simulink model "completed_microinverter_setup"  (R2022a)
settings: Solver=FixedStepDiscrete  StartTime=0.0  StopTime=2  FixedStep=Ts  RelTol=1e-3
InitFcn:
  | Ts=1e-6;
  | Tcs=1e-4;
values from neighbouring files (symbols this model uses):
  C1_filter = 2e-6    (= 2e-06)    [q4.m]
  C_filter = 100e-6    (= 0.0001)    [q1.m]    (also in q2.m; q4.m = 2e-06)
  f_center = 50    [q4.m]
  F_switch = 1e3    (= 1000)    [q1.m]
  Ki_current = L_filter*Wn^2    (= 15791.3670417)    [q1.m]    (also in q2.m = 63165.468167; q4.m = 493.480220054)
  Ki_pll = (Wn^2) / A    (= 394784.176044)    [q1.m]    (also in q4.m = 1579136.70417)
  Ki_power = 100    [q4.m]
  Ki_voltage = C_filter*Wn^2    (= 3.55305758439)    [q1.m]    (also in q4.m = 0.0710611516878)
  Kp_current = 2*L_filter*DF*Wn    (= 110.584061406)    [q1.m]    (also in q2.m = 71.0753921948; q4.m = 5.49778714378)
  Kp_pll = 2*DF / sqrt(A/Ki_pll)    [q1.m]    (also in q4.m = 2*DF / sqrt(1/Ki_pll))
  Kp_power = 0    [q4.m]
  Kp_voltage = 2*C_filter*DF*Wn    (= 0.0565486677646)    [q1.m]    (also in q4.m = 0.00791681348705)
  L1_filter = 1.5e-3    (= 0.0015)    [q4.m]
  L2_filter = 1.0e-3    (= 0.001)    [q4.m]
  L_filter = 40e-3    (= 0.04)    [q1.m]    (also in q2.m; q4.m = 0.00125)
  L_load = sqrt((R_load * V_rms^2)/P_load - R_load^2) / w    [q1.m]    (also in q4.m)
  R_load = (V_rms^2) * (pf_load^2) / P_load    (= 43.32)    [q1.m]    (also in q4.m)
  Rd_filter = 0.2    [q4.m]
  Tes = 20*Ts    (= 2e-05)    [q1.m]    (also in q4.m)
  V_dc = sqrt(2) * sqrt(3) * V_rms    [q1.m]    (also in q4.m = V_rms * sqrt(3) * sqrt(2))
undefined symbols (not defined in the file or in its folder): DiscIntNeverNeededParam
libraries: ee_lib x111, nesl_utility x28, fl_lib x23, spsabctodq0Lib x11, dspindex x3, spsTriangleGeneratorLib x2, spsdq0toabcLib x2
(part 3 of 4)

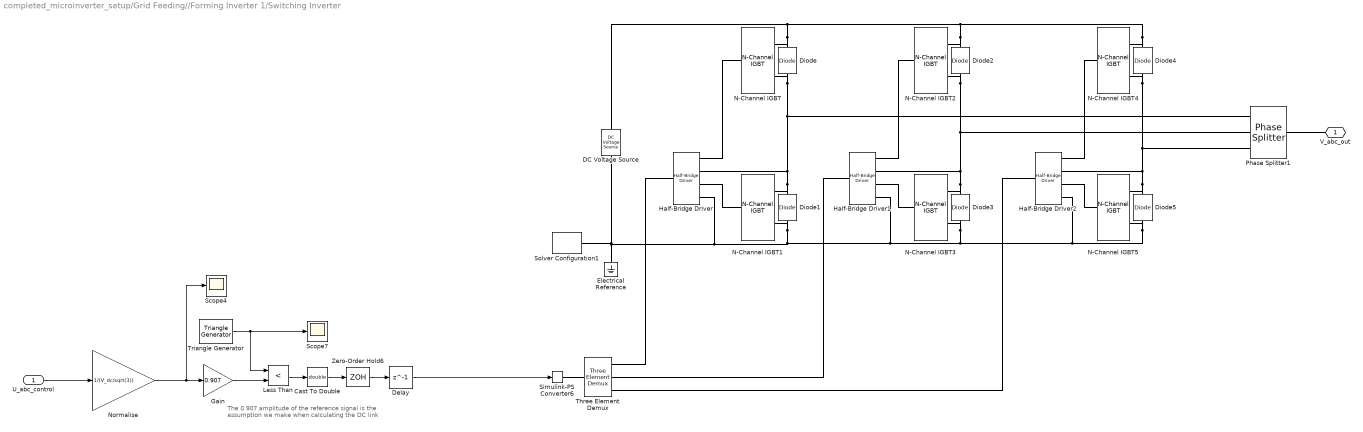
== system completed_microinverter_setup/Grid Feeding//Forming Inverter 1/Switching Inverter ==
  note: The 0.907 amplitude of the reference signal is the assumption we make when calculating the DC link
  U_abc_control : Inport
  Cast To Double : DataTypeConversion  OutDataTypeStr=double  SaturateOnIntegerOverflow=off  RndMeth=Floor
  DC Voltage Source : ee_lib/Additional Components/SPICE Sources/DC Voltage Source  DC=V_dc V
  Delay : Delay  DelayLength=1
  Diode{,1..5} (6 alike) : ee_lib/Semiconductors & Converters/Diode  ModelType=ee.enum.diode.modelType.pwl  TableType=ee.enum.diode.tableType.IfMat  IfMat=[.07, .12, .19, 1.75, 4.24, 7.32, 11.2; .16, .3, .72, 2.14, 5.02, 8.35, 13.12] A  VfMat=[.9, 1.15, 1.25, 1.5, 1.75, 2.17, 2.6, 2.85; .58, .68, .75, 1.1, 1.38, 1.77, 2.27, 2.7] V  TjVec=[25, 125] degC  VfVec=[.5, .7, .9, 1.3, 1.7, 2.1, 2.5] V  IfVec=[.1, .2, .5, 1, 2, 4, 7, 10] A  Vf=0.6 V  Ron=0.3 Ohm  Goff=1e-8 S  prmExp=ee.enum.diode.expParam.useTwo  I12=[.0137, .545] A  V12=[.6, .7] V  RS=0 Ohm  Tmeas=25 degC  IS=1e-12 A  ec=1  I1=0.0137 A  V1=0.6 V  N_series=1  N_parallel=1  Rz=0.3 Ohm  BV=inf V  C_param=ee.enum.diode.capParam.fixed  CJ=5 pF  CJ0=5 pF  Vvec=[.1, 10, 100] V  Cvec=[3.5, 1, .4] pF  VJ=1 V  Mgrad=0.5  FC=0.5  Q_param=ee.enum.diode.recoveryParam.off  iRM=-7.15 A  iF=4 A  didt=-750 A/us  trr_factor=3  trr=115 ns  Qrr=150 nA*s  Vr=-600 V  Ls=150 nH  Erec=0.03 J  TT=50 ns  tau=100 ns  T_param=ee.enum.diode.temperatureParam.off  Tdevice=25 degC  I1_T2=0.245 A  V1_T2=0.5 V  IS_T2=1.25e-7 A  Tmeas2=125 degC  XTI_param=ee.enum.diode.xtiParam.pn  XTI=3  EG_param=ee.enum.diode.egapParam.material_si  EG=1.11 eV  dBVdT=0 V/K  enable_faults=simscape.enum.onoff.off  fault_action=simscape.enum.assert.action.none  fault_types=ee.enum.diode.faults.open  tau_fault=1e-3 s  IfMat_faulted=[.07, .12, .19, 1.75, 4.24, 7.32, 11.2; .16, .3, .72, 2.14, 4.02, 6.35, 9.12] A  VfMat_faulted=[.9, 1.15, 1.25, 1.5, 1.75, 2.17, 2.6, 2.85; .58, .68, .75, 1.1, 1.38, 1.77, 2.27, 2.7] V  VfVec_faulted=[.5, .7, .9, 1.3, 1.7, 2.1, 2.5] V  IfVec_faulted=[.1, .2, .5, 1, 2, 4, 7, 10] A  Ropen_faulted=1000 Ohm  Gshort_faulted=1000 1/Ohm  Vf_faulted=0.6 V  Ron_faulted=0.3 Ohm  Goff_faulted=1e-8 S  I12_faulted=[.0137, .545] A  V12_faulted=[.6, .7] V  IS_faulted=1e-12 A  ec_faulted=1  I1_faulted=0.0137 A  V1_faulted=0.6 V  RS_faulted=0 Ohm  Rz_faulted=0.3 Ohm  BV_faulted=inf V  Cscale_faulted=100  enable_temporal_fault=simscape.enum.onoff.off  t_fault=inf s  enable_behavioral_fault=simscape.enum.onoff.off  max_permissible_voltage=inf V  n_fail_on_voltage=1  max_permissible_current=inf A  t_fail_on_current=1 s  max_permissible_dVdt=inf V/s  enable_fault_input=simscape.enum.onoff.off  i_specify=off  i_priority=None  i=0 A  i_nominal_specify=off  i_nominal_unit=A  i_nominal_value=1  v_specify=off  v_priority=None  v=0 V  v_nominal_specify=off  v_nominal_unit=V  v_nominal_value=1  i_diode_specify=off  i_diode_priority=None  i_diode=0 A  i_diode_nominal_specify=off  i_diode_nominal_unit=A  i_diode_nominal_value=1  v_diode_specify=off  v_diode_priority=None  v_diode=0 V  v_diode_nominal_specify=off  v_diode_nominal_unit=V  v_diode_nominal_value=1  i_capacitor_specify=off  i_capacitor_priority=None  i_capacitor=0 A  i_capacitor_nominal_specify=off  i_capacitor_nominal_unit=A  i_capacitor_nominal_value=1  v_capacitor_specify=off  v_capacitor_priority=None  v_capacitor=0 V  v_capacitor_nominal_specify=off  v_capacitor_nominal_unit=V  v_capacitor_nominal_value=1  power_dissipated_specify=off  power_dissipated_priority=None  power_dissipated=0 W  power_dissipated_nominal_specify=off  power_dissipated_nominal_unit=W  power_dissipated_nominal_value=1  max_permissible_temperature=inf K  t_fail_on_temperature=1 s  thermal_network_parameterization=ee.enum.thermalNetworkTopology.junctionCase  Rth=[0, 10] K/W  Rth_Cauer=[1, 3, 10] K/W  Rth_Foster=[4, 6] K/W  thermal_mass_parameterization=ee.enum.thermalNetwork.timeconstant  thermal_mass=[0, 1] J/K  thermal_mass_Cauer=[.1, .3, 1] J/K  thermal_mass_Foster=[1.5, 3] J/K  thermal_time_constant=[0, 10] s  thermal_time_constant_Cauer=[1, 3, 10] s  thermal_time_constant_Foster=[6, 18] s  thermal_mass_initial_temperatures=[25, 25] degC  thermal_mass_initial_temperatures_Cauer=[25, 25, 25] degC  steadyState_Foster=simscape.enum.onoff.on  Tvec_initial_Foster=[25, 25, 25, 25] degC
  Electrical Reference : fl_lib/Electrical/Electrical Elements/Electrical Reference
      settings: SourceProductBaseCode=PW,SS,VE
  Gain : Gain  Gain=0.907
  Half-Bridge Driver : ee_lib/Semiconductors & Converters/Half-Bridge Driver  uHighValue=0.7  uLowValue=0.3  vHigh=15 V  vLow=0 V  tpLH=50 ns  tdLH=100 ns  tpHL=50 ns  tdHL=100 ns  parameterization=1  rHigh=2 Ohm  rLow=2 Ohm  tRise=20 ns  tFall=20 ns  cLoad=10 nF  enable_faults=0  t_fault=1 s  fault_type=1  ZonTime_specify=off  ZonTime_priority=None  ZonTime=0 s  ZoffTime_specify=off  ZoffTime_priority=None  ZoffTime=0 s  power_dissipated_high_side_specify=off  power_dissipated_high_side_priority=None  power_dissipated_high_side=0 W  power_dissipated_high_side_nominal_specify=off  power_dissipated_high_side_nominal_unit=W  power_dissipated_high_side_nominal_value=1  power_dissipated_low_side_specify=off  power_dissipated_low_side_priority=None  power_dissipated_low_side=0 W  power_dissipated_low_side_nominal_specify=off  power_dissipated_low_side_nominal_unit=W  power_dissipated_low_side_nominal_value=1  uHigh=2.0 V  uLow=0.8 V
      settings: SourceProductBaseCode=PS  InternalSimscapePortConfiguration="{\"Bottom\":[],\"Left\":[{\"id\":\"u\",\"label\":\"u\",\"type\":\"input\"}],\"Right\":[{\"id\":\"HO\",\"label\":\"HO\",\"type\":\"foundation.electrical.electrical\"},{\"id\":\"HS\",\"label\":\"HS\",\"type\":\"foundation.electrical.electrical\"},{\"id\":\"LO\",\"label\":\"LO\",\"type\":\"foundation.electrical.electrical\"},{\"id\":\"LS\",\"label\":\"LS\",\"type\":\"foundation.electrical.electrical\"}],\"Top\":[]}"
  Half-Bridge Driver1 : ee_lib/Semiconductors & Converters/Half-Bridge Driver  uHighValue=0.7  uLowValue=0.3  vHigh=15 V  vLow=0 V  tpLH=50 ns  tdLH=100 ns  tpHL=50 ns  tdHL=100 ns  parameterization=1  rHigh=2 Ohm  rLow=2 Ohm  tRise=20 ns  tFall=20 ns  cLoad=10 nF  enable_faults=0  t_fault=1 s  fault_type=1  ZonTime_specify=off  ZonTime_priority=None  ZonTime=0 s  ZoffTime_specify=off  ZoffTime_priority=None  ZoffTime=0 s  power_dissipated_high_side_specify=off  power_dissipated_high_side_priority=None  power_dissipated_high_side=0 W  power_dissipated_high_side_nominal_specify=off  power_dissipated_high_side_nominal_unit=W  power_dissipated_high_side_nominal_value=1  power_dissipated_low_side_specify=off  power_dissipated_low_side_priority=None  power_dissipated_low_side=0 W  power_dissipated_low_side_nominal_specify=off  power_dissipated_low_side_nominal_unit=W  power_dissipated_low_side_nominal_value=1  uHigh=2.0 V  uLow=0.8 V
      settings: SourceProductBaseCode=PS  InternalSimscapePortConfiguration="{\"Bottom\":[],\"Left\":[{\"id\":\"u\",\"label\":\"u\",\"type\":\"input\"}],\"Right\":[{\"id\":\"HO\",\"label\":\"HO\",\"type\":\"foundation.electrical.electrical\"},{\"id\":\"HS\",\"label\":\"HS\",\"type\":\"foundation.electrical.electrical\"},{\"id\":\"LO\",\"label\":\"LO\",\"type\":\"foundation.electrical.electrical\"},{\"id\":\"LS\",\"label\":\"LS\",\"type\":\"foundation.electrical.electrical\"}],\"Top\":[]}"
  Half-Bridge Driver2 : ee_lib/Semiconductors & Converters/Half-Bridge Driver  uHighValue=0.7  uLowValue=0.3  vHigh=15 V  vLow=0 V  tpLH=50 ns  tdLH=100 ns  tpHL=50 ns  tdHL=100 ns  parameterization=1  rHigh=2 Ohm  rLow=2 Ohm  tRise=20 ns  tFall=20 ns  cLoad=10 nF  enable_faults=0  t_fault=1 s  fault_type=1  ZonTime_specify=off  ZonTime_priority=None  ZonTime=0 s  ZoffTime_specify=off  ZoffTime_priority=None  ZoffTime=0 s  power_dissipated_high_side_specify=off  power_dissipated_high_side_priority=None  power_dissipated_high_side=0 W  power_dissipated_high_side_nominal_specify=off  power_dissipated_high_side_nominal_unit=W  power_dissipated_high_side_nominal_value=1  power_dissipated_low_side_specify=off  power_dissipated_low_side_priority=None  power_dissipated_low_side=0 W  power_dissipated_low_side_nominal_specify=off  power_dissipated_low_side_nominal_unit=W  power_dissipated_low_side_nominal_value=1  uHigh=2.0 V  uLow=0.8 V
      settings: SourceProductBaseCode=PS  InternalSimscapePortConfiguration="{\"Bottom\":[],\"Left\":[{\"id\":\"u\",\"label\":\"u\",\"type\":\"input\"}],\"Right\":[{\"id\":\"HO\",\"label\":\"HO\",\"type\":\"foundation.electrical.electrical\"},{\"id\":\"HS\",\"label\":\"HS\",\"type\":\"foundation.electrical.electrical\"},{\"id\":\"LO\",\"label\":\"LO\",\"type\":\"foundation.electrical.electrical\"},{\"id\":\"LS\",\"label\":\"LS\",\"type\":\"foundation.electrical.electrical\"}],\"Top\":[]}"
  Less Than : RelationalOperator  Operator=<  OutDataTypeStr=boolean  RndMeth=Simplest  InputSameDT=off
  N-Channel IGBT{,1..5} (6 alike) : ee_lib/Semiconductors & Converters/N-Channel IGBT  model_type=ee.enum.igbt.parameterization.equation  Ices=2 mA  Vces=600 V  Vth=6 V  Vce_sat=2.6 V  Ice_sat=400 A  Vge_sat=10 V  Tmeas=25 degC  Vge_vec=[-1, 0, .5, 1, 1.5, 2, 2.5, 3, 3.5, 4] V  Vce_vec=[-2, 6, 7, 8, 10, 12, 15, 20] V  T_vec=[25, 125] degC  Ic_mat=[-1.015e-05, -9.9869e-06, -9.955e-06, -9.955e-06, -9.955e-06, -9.9549e-06, -9.9549e-06, -9.9549e-06; 1.35e-08, 1.35e-08, 1.35e-08, 1.35e-08, 1.35e-08, 1.35e-08, 1.35e-08, 1.35e-08; .00047135, .00047135, .0065225, .0065235, .006524, .0065242, .0065243, .0065244; .0005092, .0005092, 3.3324, 3.5783, 3.7206, 3.7716, 3.8067, 3.8324; .0005105, .0005105, 48.154, 70.264, 89.171, 97.793, 104.52, 109.92; .00051175, .00051175, 93.661, 166.33, 228.09, 256.21, 278.11, 295.67; .00051299, .00051299, 105.52, 252.4, 371.63, 424.27, 464.6, 496.54; .00051423, .00051423, 105.72, 317.67, 511.02, 592.92, 654.37, 702.28; .00051548, .00051548, 105.93, 353.38, 642.69, 759.2, 844.57, 909.96; .00051672, .00051672, 106.14, 357.39, 764.04, 921.52, 1033.9, 1118.3] A  Ic_mat_3D=zeros(10, 8, 2) A  C_param=ee.enum.igbt.capacitanceParam.fixedciss  C_GE=23.7 nF  C_GC=2.7 nF  C_CE=0 nF  C_ies=26.4 nF  C_res=2.7 nF  C_oes=0 nF  C_GE_vec=[25, 31, 26.5, 24.9, 25, 24.9, 24.6, 24.7, 24.8] nF  C_GC_vec=[55, 9, 5.5, 3.1, 2.5, 2.1, 1.9, 1.8, 1.7] nF  C_Vge_vec=0 V  C_CE_vec=[5, 11, 6.5, 4.9, 3.5, 2.7, 2.1, 1.7, 1.4] nF  C_ies_vec=[80, 40, 32, 28, 27.5, 27, 26.5, 26.5, 26.5] nF  C_res_vec=[55, 9, 5.5, 3.1, 2.5, 2.1, 1.9, 1.8, 1.7] nF  C_oes_vec=[60, 20, 12, 8, 6, 4.8, 4, 3.5, 3.1] nF  C_Vce_vec=[0, 1, 2, 5, 10, 15, 20, 25, 30] V  charge_linearity_param=ee.enum.igbt.cgcLinearity.constant  C_OX=20 nF  V_C_OX=-5 V  TF=0 us  TT=0 us  ec=1  VAF=200 V  RC=0.001 Ohm  RE=0.001 Ohm  RG=0.001 Ohm  BF=50  T_param=ee.enum.igbt.temperatureParameterization.none  Ices_T2=100 mA  EG=1.11 eV  Vce_sat_T2=3 V  Tmeas2=125 degC  XTI=3  BEX=-1.5  RG_alpha=0 1/K  Tdevice=300 K  Tdevice_3D=25 degC  has_thermal_port=1  thermal_network_parameterization=ee.enum.thermalNetworkTopology.junctionCase  Rth=[0, 10] K/W  Rth_Cauer=[1, 3, 10] K/W  Rth_Foster=[4, 6] K/W  thermal_mass_parameterization=ee.enum.thermalNetwork.timeconstant  thermal_mass=[0, 1] J/K  thermal_mass_Cauer=[.1, .3, 1] J/K  thermal_mass_Foster=[1.5, 3] J/K  thermal_time_constant=[0, 10] s  thermal_time_constant_Cauer=[1, 3, 10] s  thermal_time_constant_Foster=[6, 18] s  thermal_mass_initial_temperatures=[25, 25] degC  thermal_mass_initial_temperatures_Cauer=[25, 25, 25] degC  steadyState_Foster=simscape.enum.onoff.on  Tvec_initial_Foster=[25, 25, 25, 25] degC  Ic_vec1=[0, 10, 50, 100, 200, 400, 600] A  Vce_vec1=[0, 1.1, 1.3, 1.45, 1.75, 2.25, 2.7] V  Rmiller=0.1 Ohm  Goff=1e-5 1/Ohm  t_on=0.07 us  t_rise=0.7 us  t_off=0.2 us  t_fall=0.5 us  v_meas=300 V  vStartTurnOn_specify=off  vStartTurnOn_priority=None  vStartTurnOn=1 V  tStartTurnOn_specify=off  tStartTurnOn_priority=None  tStartTurnOn=0 s  vStartTurnOff_specify=off  vStartTurnOff_priority=None  vStartTurnOff=0.5 V  tStartTurnOff_specify=off  tStartTurnOff_priority=None  tStartTurnOff=0 s  Tj_vec1=[298.15, 398.15] K  Vce_mat1=[0, 1.1, 1.3, 1.45, 1.75, 2.25, 2.7; 0, 1, 1.15, 1.35, 1.7, 2.35, 3] V  Tj_vec_loss=[298.15, 398.15] K  Ic_vec_loss=[0, 10, 50, 100, 200, 400, 600] A  E_turn_on_mat1=[0, .2, 1, 2, 4, 8, 15; 0, .3, 1.3, 2.5, 5, 11, 18] * 1e-3 J  E_turn_off_mat1=[0, .3, 1.5, 3, 6, 15, 25; 0, .7, 3.3, 6.5, 13, 25, 35] * 1e-3 J  iStartTurnOff_specify=off  iStartTurnOff_priority=None  iStartTurnOff=0 A  Tdevice_specify=off  Tdevice_priority=None
      settings: SourceProductBaseCode=PS  InternalSimscapePortConfiguration="{\"Bottom\":[],\"Left\":[{\"id\":\"G\",\"label\":\"\",\"type\":\"foundation.electrical.electrical\"}],\"Right\":[{\"id\":\"C\",\"label\":\"\",\"type\":\"foundation.electrical.electrical\"},{\"id\":\"E\",\"label\":\"\",\"type\":\"foundation.electrical.electrical\"}],\"Top\":[]}"
  Normalise : Gain  Gain=1/(V_dc/sqrt(3))
  Phase Splitter1 : ee_lib/Connectors & References/Phase Splitter
      settings: SourceProductBaseCode=PS
  Scope4 : Scope
  Scope7 : Scope
  Simulink-PS Converter6 : nesl_utility/Simulink-PS Converter  PhysicalDomain=network_engine_domain  SubClassName=ps_input  LeftPortType=input  RightPortType=output  PseudoPeriodic=off  Frequencies=[]  NoiseDistribution=none  NoiseParameters=[]  Unit=1  AffineConversion=off  FilteringAndDerivatives=provide  SimscapeFilterOrder=1  InputFilterTimeConstant=0.001  UdotUserProvided=0
      settings: SourceProductBaseCode=SS,PW,VE
  Solver Configuration1 : nesl_utility/Solver Configuration  PhysicalDomain=network_engine_domain  SubClassName=solver  LeftPortType=input  RightPortType=generic  Tones=[]  Harmonics=[]  SimulateNoise=off  Profile=off  UseLocalSampling=off  EnableSwitchedLinearOptims=on  FrequencyDomain=off  UseCCode=off  RelTol=0.001  AbsTol=1e-06  MinStep=1e-09  ToWorkspace=off  RevertToSquareIcSolve=off  NumHomotopyIterations=100  PhasorMode=off  PhasorModeNumHarmonics=1  IndexReductionMethod=DerivativeReplacement  DoDC=off  ResidualTolerance=1e-09  UseLocalSolver=on  LocalSolverChoice=NE_BACKWARD_EULER_ADVANCER  LocalSolverSampleTime=Ts  DoFixedCost=off  MaxNonlinIter=3  MaxModeIter=2  ComputeImpulses=off  ImpulseIterations=2  LinearAlgebra=auto  LinearAlgebraNumThread=0  EquationFormulation=NE_TIME_EF  DelaysMemoryBudget=1024  AutomaticFiltering=off  FilteringTimeConstant=0.001  PartitionStorageMethod=AS_NEEDED  PartitionMemoryBudget=1024  PartitionMethod=ROBUST
      settings: SourceProductBaseCode=SS,PW,VE
  Three Element Demux : ee_lib/Connectors & References/Three Element Demux
      settings: SourceProductBaseCode=PS  InternalSimscapePortConfiguration="{\"Bottom\":[],\"Left\":[{\"id\":\"abc\",\"label\":\"abc\",\"type\":\"input\"}],\"Right\":[{\"id\":\"a\",\"label\":\"a\",\"type\":\"output\"},{\"id\":\"b\",\"label\":\"b\",\"type\":\"output\"},{\"id\":\"c\",\"label\":\"c\",\"type\":\"output\"}],\"Top\":[]}"
  Triangle Generator : spsTriangleGeneratorLib/Triangle Generator  Freq=F_switch  Phase=0  Ts=Ts
  Zero-Order Hold6 : ZeroOrderHold  SampleTime=Ts
  V_abc_out : PMIOPort  Side=Right
  wires:
  Triangle Generator/1 -> Scope7/1, Less Than/1
  Gain/1 -> Less Than/2
  Normalise/1 -> Scope4/1, Gain/1
  Less Than/1 -> Cast To Double/1
  Cast To Double/1 -> Zero-Order Hold6/1
  U_abc_control/1 -> Normalise/1
  Zero-Order Hold6/1 -> Delay/1
  Delay/1 -> Simulink-PS Converter6/1
  connections:
  N-Channel IGBT1/RConn2 -- Half-Bridge Driver1/RConn4 -- Half-Bridge Driver2/RConn4 -- N-Channel IGBT5/RConn2 -- Diode5/LConn1 -- N-Channel IGBT3/RConn2 -- Diode3/LConn1 -- Half-Bridge Driver/RConn4 -- Solver Configuration1/RConn1 -- DC Voltage Source/RConn1 -- Electrical Reference/LConn1 -- Diode1/LConn1
  Half-Bridge Driver1/RConn2 -- Phase Splitter1/RConn2 -- N-Channel IGBT2/RConn2 -- Diode2/LConn1 -- Diode3/RConn1 -- N-Channel IGBT3/RConn1
  Phase Splitter1/RConn3 -- Half-Bridge Driver2/RConn2 -- N-Channel IGBT5/RConn1 -- Diode5/RConn1 -- Diode4/LConn1 -- N-Channel IGBT4/RConn2
  Diode/LConn1 -- Phase Splitter1/RConn1 -- Half-Bridge Driver/RConn2 -- N-Channel IGBT1/RConn1 -- Diode1/RConn1 -- N-Channel IGBT/RConn2
  Diode/RConn1 -- N-Channel IGBT/RConn1 -- N-Channel IGBT4/RConn1 -- Diode4/RConn1 -- N-Channel IGBT2/RConn1 -- Diode2/RConn1 -- DC Voltage Source/LConn1
  Half-Bridge Driver/RConn3 -- N-Channel IGBT1/LConn1
  Three Element Demux/RConn3 -- Half-Bridge Driver2/LConn1
  N-Channel IGBT5/LConn1 -- Half-Bridge Driver2/RConn3
  Half-Bridge Driver/RConn1 -- N-Channel IGBT/LConn1
  Three Element Demux/RConn2 -- Half-Bridge Driver1/LConn1
  Three Element Demux/LConn1 -- Simulink-PS Converter6/RConn1
  N-Channel IGBT3/LConn1 -- Half-Bridge Driver1/RConn3
  Three Element Demux/RConn1 -- Half-Bridge Driver/LConn1
  N-Channel IGBT2/LConn1 -- Half-Bridge Driver1/RConn1
  N-Channel IGBT4/LConn1 -- Half-Bridge Driver2/RConn1
  V_abc_out/RConn1 -- Phase Splitter1/LConn1

== system completed_microinverter_setup/Grid Feeding//Forming Inverter 2/3 Phase Grid Sensor ==
  Neutral Port (Three-Phase) : ee_lib/Connectors & References/Neutral Port (Three-Phase)  G_parasitic=1e-12 1/Ohm
      settings: SourceProductBaseCode=PS  InternalSimscapePortConfiguration="{\"Bottom\":[],\"Left\":[{\"id\":\"N\",\"label\":\"~\",\"type\":\"foundation.electrical.three_phase\"}],\"Right\":[{\"id\":\"n\",\"label\":\"n\",\"type\":\"foundation.electrical.electrical\"}],\"Top\":[]}"
  PS-Simulink Converter : nesl_utility/PS-Simulink Converter  PhysicalDomain=network_engine_domain  SubClassName=ps_output  LeftPortType=input  RightPortType=output  PseudoPeriodic=off  Frequencies=[]  VectorFormat=inherit  Unit=inherit  AffineConversion=off
      settings: SourceProductBaseCode=SS,PW,VE
  Phase Splitter1 : ee_lib/Connectors & References/Phase Splitter
      settings: SourceProductBaseCode=PS
  Phase Voltage Sensor (Three-Phase) : ee_lib/Sensors & Transducers/Phase Voltage Sensor (Three-Phase)
      settings: SourceProductBaseCode=PS
  Resistor : ee_lib/Passive/Resistor  R=R Ohm  enable_R_tol=0  R_tol=5  tol_distribution=1  nSigma=4  enable_operating_limits=0  operating_limit_action=2  max_working_voltage=100 V  power_rating=1 W  enable_faults=0  fault_action=1  R_faulted=inf Ohm  enable_temporal_fault=0  t_fault=1 s  enable_behavioral_fault=0  max_permissible_current=1 A  t_fail_on_current=1 s  noise_mode=0  sample_time=1e-3 s  repeatability=1  auto_seed=676943032  user_seed=0  Tdevice=25 degC  power_derating_T1=70 degC  power_derating_T2=155 degC  operating_temperature_range_vec=[-50, 150] degC  alpha=3.93e-3 1/K  Tmeas=25 degC  thermal_mass=100 J/K  temperature_specify=off  temperature_priority=High  temperature=298.15 K  temperature_nominal_specify=off  temperature_nominal_unit=K  temperature_nominal_value=1
  Resistor1 : ee_lib/Passive/Resistor  R=R Ohm  enable_R_tol=0  R_tol=5  tol_distribution=1  nSigma=4  enable_operating_limits=0  operating_limit_action=2  max_working_voltage=100 V  power_rating=1 W  enable_faults=0  fault_action=1  R_faulted=inf Ohm  enable_temporal_fault=0  t_fault=1 s  enable_behavioral_fault=0  max_permissible_current=1 A  t_fail_on_current=1 s  noise_mode=0  sample_time=1e-3 s  repeatability=1  auto_seed=4168664255  user_seed=0  Tdevice=25 degC  power_derating_T1=70 degC  power_derating_T2=155 degC  operating_temperature_range_vec=[-50, 150] degC  alpha=3.93e-3 1/K  Tmeas=25 degC  thermal_mass=100 J/K  temperature_specify=off  temperature_priority=High  temperature=298.15 K  temperature_nominal_specify=off  temperature_nominal_unit=K  temperature_nominal_value=1
  Resistor2 : ee_lib/Passive/Resistor  R=R Ohm  enable_R_tol=0  R_tol=5  tol_distribution=1  nSigma=4  enable_operating_limits=0  operating_limit_action=2  max_working_voltage=100 V  power_rating=1 W  enable_faults=0  fault_action=1  R_faulted=inf Ohm  enable_temporal_fault=0  t_fault=1 s  enable_behavioral_fault=0  max_permissible_current=1 A  t_fail_on_current=1 s  noise_mode=0  sample_time=1e-3 s  repeatability=1  auto_seed=4111000739  user_seed=0  Tdevice=25 degC  power_derating_T1=70 degC  power_derating_T2=155 degC  operating_temperature_range_vec=[-50, 150] degC  alpha=3.93e-3 1/K  Tmeas=25 degC  thermal_mass=100 J/K  temperature_specify=off  temperature_priority=High  temperature=298.15 K  temperature_nominal_specify=off  temperature_nominal_unit=K  temperature_nominal_value=1
  V_abc : PMIOPort  Side=Left
  V_abc_sense : Outport
  wires:
  PS-Simulink Converter/1 -> V_abc_sense/1
  connections:
  Resistor2/LConn1 -- Phase Splitter1/RConn3
  Resistor/RConn1 -- Neutral Port (Three-Phase)/RConn1 -- Resistor2/RConn1 -- Resistor1/RConn1
  Phase Splitter1/RConn2 -- Resistor1/LConn1
  Phase Splitter1/RConn1 -- Resistor/LConn1
  V_abc/RConn1 -- Phase Voltage Sensor (Three-Phase)/LConn1 -- Phase Splitter1/LConn1
  Phase Voltage Sensor (Three-Phase)/RConn2 -- Neutral Port (Three-Phase)/LConn1
  PS-Simulink Converter/LConn1 -- Phase Voltage Sensor (Three-Phase)/RConn1

== system completed_microinverter_setup/Grid Feeding//Forming Inverter 2/Calculate PQ of output ==
  note: Reorient Vdq0 so that Uq = 0, Ud = defined
  Vdq0 : Inport
  Idq0 : Inport  Port=2
  Atan2 : Trigonometry  Operator=atan2
  Cos : Trigonometry  Operator=cos
  Demux : Demux  Outputs=3
  Demux1 : Demux  Outputs=2
  Gain2 : Gain  Gain=3/2
  MatrixMultiply1 : Product  Multiplication=Matrix(*)
  MatrixMultiply2 : Product  Multiplication=Matrix(*)
  Mux : Mux
  Product : Product
  Product2 : Product
  Selector : Selector  InputPortWidth=3  IndexOptions=Index vector (dialog)  Indices=[1 2]  OutputSizes=1
  Selector1 : Selector  InputPortWidth=3  IndexOptions=Index vector (dialog)  Indices=[1]  OutputSizes=1
  Sign : Signum
  Sqrt : Sqrt
  Square : Math  Operator=square
  Subsystem : Subsystem
  Sum of Elements : Sum  Inputs=+
  Terminator : Terminator
  PQ Stats : Outport
  wires:
  Product2/1 -> Gain2/1
  Square/1 -> Sum of Elements/1
  Gain2/1 -> Demux/1, Selector/1
  Sum of Elements/1 -> Sqrt/1
  Selector/1 -> Square/1, Demux1/1
  Vdq0/1 -> MatrixMultiply1/2, Subsystem/1(Vdq0)
  Subsystem/1(Rotation Matrix) -> MatrixMultiply2/1, MatrixMultiply1/1
  Idq0/1 -> MatrixMultiply2/2
  MatrixMultiply1/1 -> Selector1/1
  MatrixMultiply2/1 -> Product2/2
  Demux/3 -> Terminator/1
  Demux/2 -> Atan2/1  "Q"
  Demux/1 -> Atan2/2  "P"
  Atan2/1 -> Cos/1
  Demux1/1 -> Mux/1  "P"
  Demux1/2 -> Sign/1, Mux/2  "Q"
  Sqrt/1 -> Mux/3  "|S|"
  Product/1 -> Mux/4  "pf"
  Mux/1 -> PQ Stats/1
  Selector1/1 -> Product2/1
  Sign/1 -> Product/1
  Cos/1 -> Product/2  "pf"

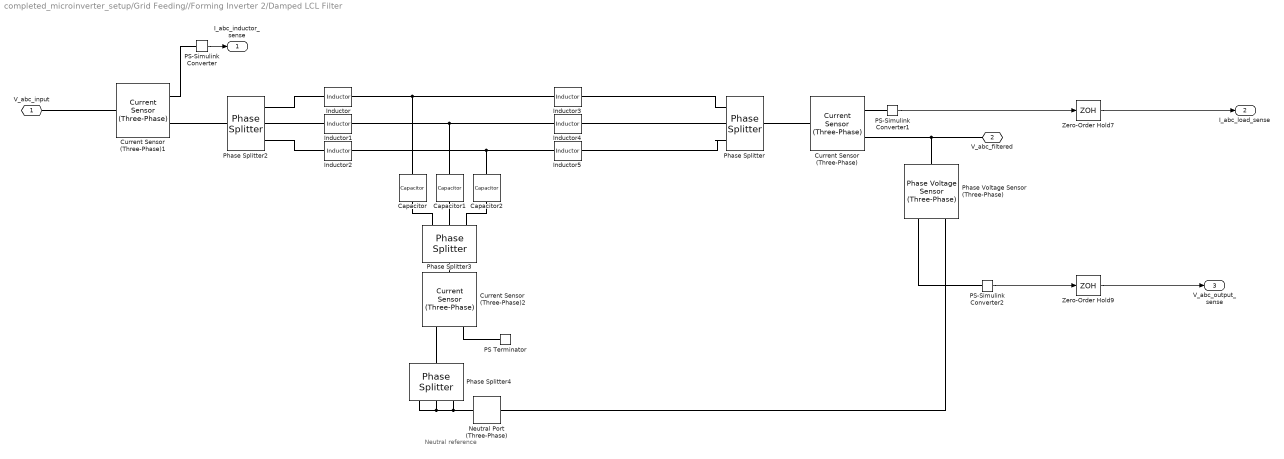
== system completed_microinverter_setup/Grid Feeding//Forming Inverter 2/Damped LCL Filter ==
  note: Neutral reference
  Capacitor : fl_lib/Electrical/Electrical Elements/Capacitor  c=C F  r=Rd Ohm  g=0 1/Ohm  i_specify=off  i_priority=None  i=0 A  i_nominal_specify=off  i_nominal_unit=A  i_nominal_value=1  v_specify=off  v_priority=None  v=0 V  v_nominal_specify=off  v_nominal_unit=V  v_nominal_value=1  vc_specify=off  vc_priority=High  vc=0 V  vc_nominal_specify=off  vc_nominal_unit=V  vc_nominal_value=1
      settings: SourceProductBaseCode=PW,SS,VE
  Capacitor1 : fl_lib/Electrical/Electrical Elements/Capacitor  c=C F  r=Rd Ohm  g=0 1/Ohm  i_specify=off  i_priority=None  i=0 A  i_nominal_specify=off  i_nominal_unit=A  i_nominal_value=1  v_specify=off  v_priority=None  v=0 V  v_nominal_specify=off  v_nominal_unit=V  v_nominal_value=1  vc_specify=off  vc_priority=High  vc=0 V  vc_nominal_specify=off  vc_nominal_unit=V  vc_nominal_value=1
      settings: SourceProductBaseCode=PW,SS,VE
  Capacitor2 : fl_lib/Electrical/Electrical Elements/Capacitor  c=C F  r=Rd Ohm  g=0 1/Ohm  i_specify=off  i_priority=None  i=0 A  i_nominal_specify=off  i_nominal_unit=A  i_nominal_value=1  v_specify=off  v_priority=None  v=0 V  v_nominal_specify=off  v_nominal_unit=V  v_nominal_value=1  vc_specify=off  vc_priority=High  vc=0 V  vc_nominal_specify=off  vc_nominal_unit=V  vc_nominal_value=1
      settings: SourceProductBaseCode=PW,SS,VE
  Current Sensor (Three-Phase) : ee_lib/Sensors & Transducers/Current Sensor (Three-Phase)
  Current Sensor (Three-Phase)1 : ee_lib/Sensors & Transducers/Current Sensor (Three-Phase)
  Current Sensor (Three-Phase)2 : ee_lib/Sensors & Transducers/Current Sensor (Three-Phase)
  Inductor : ee_lib/Passive/Inductor  l=L1 H  enable_L_tol=0  L_tol=20  tol_distribution=1  nSigma=4  r=0 Ohm  g=1e-9 1/Ohm  enable_operating_limits=0  operating_limit_action=2  max_working_current=1 A  power_rating=1 W  enable_faults=0  fault_action=1  lambdaPercent=50  k_faulted=0.9999  turnsShort=0  openCct=0  groundShort=0  groundShortG=0 1/Ohm  tau_fault=1e-3 s  enable_temporal_fault=0  t_fault=1 s  enable_behavioral_fault=0  max_permissible_voltage=100 V  n_fail_on_voltage=1  max_permissible_current=1 A  t_fail_on_current=1 s  i_L_specify=off  i_L_priority=High  i_L=0 A  i_L_nominal_specify=off  i_L_nominal_unit=A  i_L_nominal_value=1
  Inductor1 : ee_lib/Passive/Inductor  l=L1 H  enable_L_tol=0  L_tol=20  tol_distribution=1  nSigma=4  r=0 Ohm  g=1e-9 1/Ohm  enable_operating_limits=0  operating_limit_action=2  max_working_current=1 A  power_rating=1 W  enable_faults=0  fault_action=1  lambdaPercent=50  k_faulted=0.9999  turnsShort=0  openCct=0  groundShort=0  groundShortG=0 1/Ohm  tau_fault=1e-3 s  enable_temporal_fault=0  t_fault=1 s  enable_behavioral_fault=0  max_permissible_voltage=100 V  n_fail_on_voltage=1  max_permissible_current=1 A  t_fail_on_current=1 s  i_L_specify=off  i_L_priority=High  i_L=0 A  i_L_nominal_specify=off  i_L_nominal_unit=A  i_L_nominal_value=1
  Inductor2 : ee_lib/Passive/Inductor  l=L1 H  enable_L_tol=0  L_tol=20  tol_distribution=1  nSigma=4  r=0 Ohm  g=1e-9 1/Ohm  enable_operating_limits=0  operating_limit_action=2  max_working_current=1 A  power_rating=1 W  enable_faults=0  fault_action=1  lambdaPercent=50  k_faulted=0.9999  turnsShort=0  openCct=0  groundShort=0  groundShortG=0 1/Ohm  tau_fault=1e-3 s  enable_temporal_fault=0  t_fault=1 s  enable_behavioral_fault=0  max_permissible_voltage=100 V  n_fail_on_voltage=1  max_permissible_current=1 A  t_fail_on_current=1 s  i_L_specify=off  i_L_priority=High  i_L=0 A  i_L_nominal_specify=off  i_L_nominal_unit=A  i_L_nominal_value=1
  Inductor3 : ee_lib/Passive/Inductor  l=L2 H  enable_L_tol=0  L_tol=20  tol_distribution=1  nSigma=4  r=0 Ohm  g=1e-9 1/Ohm  enable_operating_limits=0  operating_limit_action=2  max_working_current=1 A  power_rating=1 W  enable_faults=0  fault_action=1  lambdaPercent=50  k_faulted=0.9999  turnsShort=0  openCct=0  groundShort=0  groundShortG=0 1/Ohm  tau_fault=1e-3 s  enable_temporal_fault=0  t_fault=1 s  enable_behavioral_fault=0  max_permissible_voltage=100 V  n_fail_on_voltage=1  max_permissible_current=1 A  t_fail_on_current=1 s  i_L_specify=off  i_L_priority=High  i_L=0 A  i_L_nominal_specify=off  i_L_nominal_unit=A  i_L_nominal_value=1
  Inductor4 : ee_lib/Passive/Inductor  l=L2 H  enable_L_tol=0  L_tol=20  tol_distribution=1  nSigma=4  r=0 Ohm  g=1e-9 1/Ohm  enable_operating_limits=0  operating_limit_action=2  max_working_current=1 A  power_rating=1 W  enable_faults=0  fault_action=1  lambdaPercent=50  k_faulted=0.9999  turnsShort=0  openCct=0  groundShort=0  groundShortG=0 1/Ohm  tau_fault=1e-3 s  enable_temporal_fault=0  t_fault=1 s  enable_behavioral_fault=0  max_permissible_voltage=100 V  n_fail_on_voltage=1  max_permissible_current=1 A  t_fail_on_current=1 s  i_L_specify=off  i_L_priority=High  i_L=0 A  i_L_nominal_specify=off  i_L_nominal_unit=A  i_L_nominal_value=1
  Inductor5 : ee_lib/Passive/Inductor  l=L2 H  enable_L_tol=0  L_tol=20  tol_distribution=1  nSigma=4  r=0 Ohm  g=1e-9 1/Ohm  enable_operating_limits=0  operating_limit_action=2  max_working_current=1 A  power_rating=1 W  enable_faults=0  fault_action=1  lambdaPercent=50  k_faulted=0.9999  turnsShort=0  openCct=0  groundShort=0  groundShortG=0 1/Ohm  tau_fault=1e-3 s  enable_temporal_fault=0  t_fault=1 s  enable_behavioral_fault=0  max_permissible_voltage=100 V  n_fail_on_voltage=1  max_permissible_current=1 A  t_fail_on_current=1 s  i_L_specify=off  i_L_priority=High  i_L=0 A  i_L_nominal_specify=off  i_L_nominal_unit=A  i_L_nominal_value=1
  Neutral Port (Three-Phase) : ee_lib/Connectors & References/Neutral Port (Three-Phase)  G_parasitic=1e-12 1/Ohm
      settings: SourceProductBaseCode=PS  InternalSimscapePortConfiguration="{\"Bottom\":[],\"Left\":[{\"id\":\"N\",\"label\":\"~\",\"type\":\"foundation.electrical.three_phase\"}],\"Right\":[{\"id\":\"n\",\"label\":\"n\",\"type\":\"foundation.electrical.electrical\"}],\"Top\":[]}"
  PS Terminator : fl_lib/Physical Signals/Sinks/PS Terminator
      settings: SourceProductBaseCode=PW,SS,VE
  PS-Simulink Converter : nesl_utility/PS-Simulink Converter  PhysicalDomain=network_engine_domain  SubClassName=ps_output  LeftPortType=input  RightPortType=output  PseudoPeriodic=off  Frequencies=[]  VectorFormat=inherit  Unit=inherit  AffineConversion=off
      settings: SourceProductBaseCode=SS,PW,VE
  PS-Simulink Converter1 : nesl_utility/PS-Simulink Converter  PhysicalDomain=network_engine_domain  SubClassName=ps_output  LeftPortType=input  RightPortType=output  PseudoPeriodic=off  Frequencies=[]  VectorFormat=inherit  Unit=inherit  AffineConversion=off
      settings: SourceProductBaseCode=SS,PW,VE
  PS-Simulink Converter2 : nesl_utility/PS-Simulink Converter  PhysicalDomain=network_engine_domain  SubClassName=ps_output  LeftPortType=input  RightPortType=output  PseudoPeriodic=off  Frequencies=[]  VectorFormat=inherit  Unit=inherit  AffineConversion=off
      settings: SourceProductBaseCode=SS,PW,VE
  Phase Splitter{,2..4} (4 alike) : ee_lib/Connectors & References/Phase Splitter
      settings: SourceProductBaseCode=PS
  Phase Voltage Sensor (Three-Phase) : ee_lib/Sensors & Transducers/Phase Voltage Sensor (Three-Phase)
      settings: SourceProductBaseCode=PS
  Zero-Order Hold7 : ZeroOrderHold  SampleTime=Ts
  Zero-Order Hold9 : ZeroOrderHold  SampleTime=Ts
  V_abc_input : PMIOPort  Side=Left
  V_abc_filtered : PMIOPort  Port=2  Side=Right
  I_abc_inductor_sense : Outport
  I_abc_load_sense : Outport  Port=2
  V_abc_output_sense : Outport  Port=3
  wires:
  PS-Simulink Converter/1 -> I_abc_inductor_sense/1
  PS-Simulink Converter1/1 -> Zero-Order Hold7/1
  Zero-Order Hold7/1 -> I_abc_load_sense/1
  PS-Simulink Converter2/1 -> Zero-Order Hold9/1
  Zero-Order Hold9/1 -> V_abc_output_sense/1
  connections:
  Capacitor1/LConn1 -- Inductor4/LConn1 -- Inductor1/RConn1
  Capacitor/LConn1 -- Inductor3/LConn1 -- Inductor/RConn1
  Capacitor2/LConn1 -- Inductor5/LConn1 -- Inductor2/RConn1
  Phase Voltage Sensor (Three-Phase)/LConn1 -- Current Sensor (Three-Phase)/RConn2 -- V_abc_filtered/RConn1
  Phase Voltage Sensor (Three-Phase)/RConn2 -- Neutral Port (Three-Phase)/LConn1
  Current Sensor (Three-Phase)/LConn1 -- Phase Splitter/LConn1
  Phase Splitter2/RConn2 -- Inductor1/LConn1
  Phase Splitter2/RConn1 -- Inductor/LConn1
  Phase Splitter2/RConn3 -- Inductor2/LConn1
  Phase Splitter2/LConn1 -- Current Sensor (Three-Phase)1/RConn2
  PS-Simulink Converter/LConn1 -- Current Sensor (Three-Phase)1/RConn1
  PS-Simulink Converter1/LConn1 -- Current Sensor (Three-Phase)/RConn1
  PS-Simulink Converter2/LConn1 -- Phase Voltage Sensor (Three-Phase)/RConn1
  Phase Splitter3/RConn1 -- Capacitor/RConn1
  Phase Splitter3/RConn2 -- Capacitor1/RConn1
  Phase Splitter3/RConn3 -- Capacitor2/RConn1
  Phase Splitter3/LConn1 -- Current Sensor (Three-Phase)2/LConn1
  Phase Splitter4/LConn1 -- Current Sensor (Three-Phase)2/RConn2
  Phase Splitter4/RConn1 -- Neutral Port (Three-Phase)/RConn1 -- Phase Splitter4/RConn3 -- Phase Splitter4/RConn2
  V_abc_input/RConn1 -- Current Sensor (Three-Phase)1/LConn1
  Phase Splitter/RConn1 -- Inductor3/RConn1
  Phase Splitter/RConn2 -- Inductor4/RConn1
  Phase Splitter/RConn3 -- Inductor5/RConn1
  PS Terminator/LConn1 -- Current Sensor (Three-Phase)2/RConn1

== system completed_microinverter_setup/Grid Feeding//Forming Inverter 2/Ideal Inverter ==
  U_abc_control : Inport
  Controlled Voltage Source : fl_lib/Electrical/Electrical Sources/Controlled Voltage Source
      settings: SourceProductBaseCode=PW,SS,VE
  Controlled Voltage Source1 : fl_lib/Electrical/Electrical Sources/Controlled Voltage Source
      settings: SourceProductBaseCode=PW,SS,VE
  Controlled Voltage Source2 : fl_lib/Electrical/Electrical Sources/Controlled Voltage Source
      settings: SourceProductBaseCode=PW,SS,VE
  Delay : Delay  DelayLength=1
  Demux : Demux  Outputs=3
  Electrical Reference : fl_lib/Electrical/Electrical Elements/Electrical Reference
      settings: SourceProductBaseCode=PW,SS,VE
  Phase Splitter : ee_lib/Connectors & References/Phase Splitter
      settings: SourceProductBaseCode=PS
  Simulink-PS Converter3 : nesl_utility/Simulink-PS Converter  PhysicalDomain=network_engine_domain  SubClassName=ps_input  LeftPortType=input  RightPortType=output  PseudoPeriodic=off  Frequencies=[]  NoiseDistribution=none  NoiseParameters=[]  Unit=1  AffineConversion=off  FilteringAndDerivatives=provide  SimscapeFilterOrder=1  InputFilterTimeConstant=0.001  UdotUserProvided=0
      settings: SourceProductBaseCode=SS,PW,VE
  Simulink-PS Converter4 : nesl_utility/Simulink-PS Converter  PhysicalDomain=network_engine_domain  SubClassName=ps_input  LeftPortType=input  RightPortType=output  PseudoPeriodic=off  Frequencies=[]  NoiseDistribution=none  NoiseParameters=[]  Unit=1  AffineConversion=off  FilteringAndDerivatives=provide  SimscapeFilterOrder=1  InputFilterTimeConstant=0.001  UdotUserProvided=0
      settings: SourceProductBaseCode=SS,PW,VE
  Simulink-PS Converter5 : nesl_utility/Simulink-PS Converter  PhysicalDomain=network_engine_domain  SubClassName=ps_input  LeftPortType=input  RightPortType=output  PseudoPeriodic=off  Frequencies=[]  NoiseDistribution=none  NoiseParameters=[]  Unit=1  AffineConversion=off  FilteringAndDerivatives=provide  SimscapeFilterOrder=1  InputFilterTimeConstant=0.001  UdotUserProvided=0
      settings: SourceProductBaseCode=SS,PW,VE
  Zero-Order Hold6 : ZeroOrderHold  SampleTime=Tcs
  V_abc_out : PMIOPort  Side=Right
  wires:
  Demux/1 -> Simulink-PS Converter3/1
  Demux/2 -> Simulink-PS Converter4/1
  Demux/3 -> Simulink-PS Converter5/1
  Zero-Order Hold6/1 -> Delay/1
  Delay/1 -> Demux/1
  U_abc_control/1 -> Zero-Order Hold6/1
  connections:
  Phase Splitter/RConn1 -- Controlled Voltage Source/LConn1
  Phase Splitter/RConn3 -- Controlled Voltage Source2/LConn1
  Simulink-PS Converter5/RConn1 -- Controlled Voltage Source2/RConn1
  Electrical Reference/LConn1 -- Controlled Voltage Source/RConn2 -- Controlled Voltage Source1/RConn2 -- Controlled Voltage Source2/RConn2
  Phase Splitter/RConn2 -- Controlled Voltage Source1/LConn1
  Simulink-PS Converter3/RConn1 -- Controlled Voltage Source/RConn1
  Simulink-PS Converter4/RConn1 -- Controlled Voltage Source1/RConn1
  Phase Splitter/LConn1 -- V_abc_out/RConn1

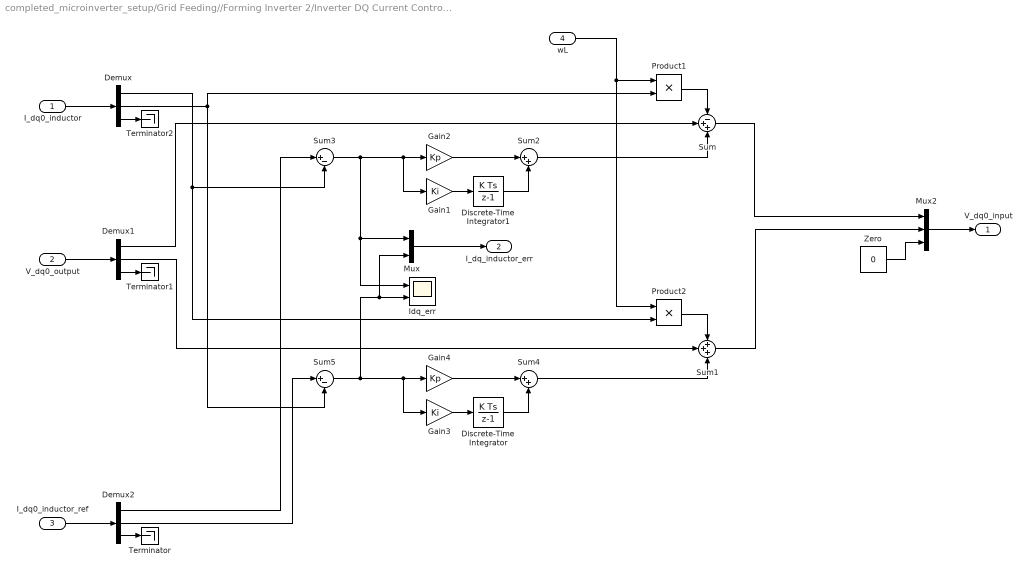
== system completed_microinverter_setup/Grid Feeding//Forming Inverter 2/Inverter DQ Current Controller ==
  I_dq0_inductor : Inport
  V_dq0_output : Inport  Port=2
  I_dq0_inductor_ref : Inport  Port=3
  wL : Inport  Port=4
  Demux : Demux  Outputs=3
  Demux1 : Demux  Outputs=3
  Demux2 : Demux  Outputs=3
  Discrete-Time Integrator : DiscreteIntegrator  SampleTime=Ts  ICPrevOutput=DiscIntNeverNeededParam  ICPrevScaledInput=DiscIntNeverNeededParam
  Discrete-Time Integrator1 : DiscreteIntegrator  SampleTime=Ts  ICPrevOutput=DiscIntNeverNeededParam  ICPrevScaledInput=DiscIntNeverNeededParam
  Gain1 : Gain  Gain=Ki
  Gain2 : Gain  Gain=Kp
  Gain3 : Gain  Gain=Ki
  Gain4 : Gain  Gain=Kp
  Idq_err : Scope  NumInputPorts=2
  Mux : Mux  Inputs=2
  Mux2 : Mux  Inputs=3
  Product1 : Product
  Product2 : Product
  Sum : Sum  Inputs=-++
  Sum1 : Sum  Inputs=+++
  Sum2 : Sum  Inputs=|++
  Sum3 : Sum  Inputs=|+-
  Sum4 : Sum  Inputs=|++
  Sum5 : Sum  Inputs=|+-
  Terminator : Terminator
  Terminator1 : Terminator
  Terminator2 : Terminator
  Zero : Constant  Value=0  OutDataTypeStr=Inherit: Inherit via back propagation
  V_dq0_input : Outport
  I_dq_inductor_err : Outport  Port=2
  wires:
  Gain3/1 -> Discrete-Time Integrator/1
  I_dq0_inductor_ref/1 -> Demux2/1
  V_dq0_output/1 -> Demux1/1
  Demux2/1 -> Sum3/1
  Discrete-Time Integrator1/1 -> Sum2/2
  Gain4/1 -> Sum4/1
  Product2/1 -> Sum1/1
  Sum5/1 -> Mux/2, Idq_err/2, Gain4/1, Gain3/1
  Mux2/1 -> V_dq0_input/1
  Demux/2 -> Sum5/2, Product1/2
  Demux/1 -> Sum3/2, Product2/2
  Demux2/3 -> Terminator/1
  I_dq0_inductor/1 -> Demux/1
  Sum/1 -> Mux2/1
  Demux1/1 -> Sum/2
  Discrete-Time Integrator/1 -> Sum4/2
  Product1/1 -> Sum/1
  Gain2/1 -> Sum2/1
  Sum2/1 -> Sum/3
  Gain1/1 -> Discrete-Time Integrator1/1
  Sum1/1 -> Mux2/2
  Zero/1 -> Mux2/3
  Sum4/1 -> Sum1/3
  Demux1/2 -> Sum1/2
  Demux2/2 -> Sum5/1
  Demux1/3 -> Terminator1/1
  Demux/3 -> Terminator2/1
  wL/1 -> Product2/1, Product1/1
  Sum3/1 -> Mux/1, Idq_err/1, Gain2/1, Gain1/1
  Mux/1 -> I_dq_inductor_err/1

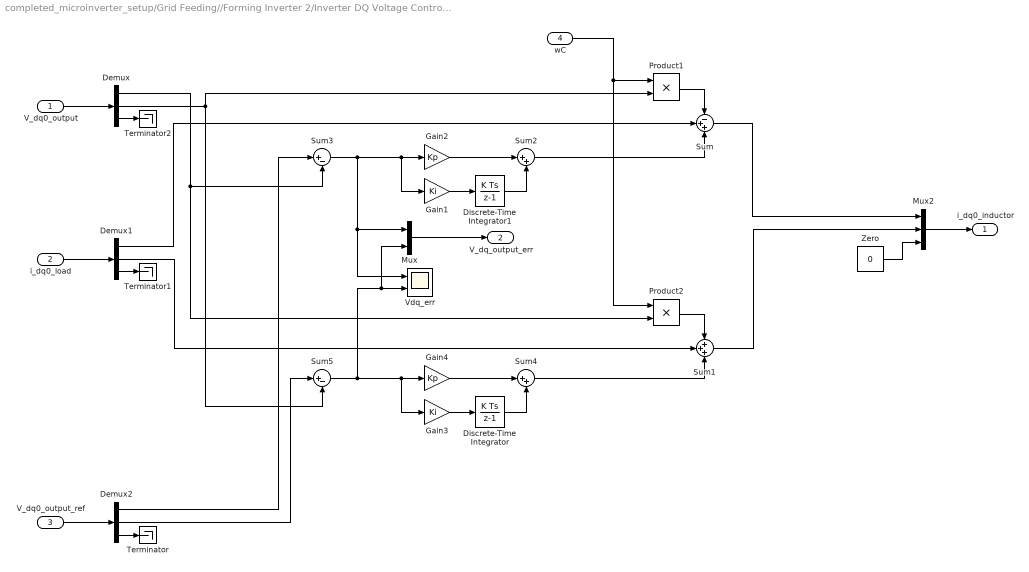
== system completed_microinverter_setup/Grid Feeding//Forming Inverter 2/Inverter DQ Voltage Controller ==
  V_dq0_output : Inport
  i_dq0_load : Inport  Port=2
  V_dq0_output_ref : Inport  Port=3
  wC : Inport  Port=4
  Demux : Demux  Outputs=3
  Demux1 : Demux  Outputs=3
  Demux2 : Demux  Outputs=3
  Discrete-Time Integrator : DiscreteIntegrator  SampleTime=Ts  ICPrevOutput=DiscIntNeverNeededParam  ICPrevScaledInput=DiscIntNeverNeededParam
  Discrete-Time Integrator1 : DiscreteIntegrator  SampleTime=Ts  ICPrevOutput=DiscIntNeverNeededParam  ICPrevScaledInput=DiscIntNeverNeededParam
  Gain1 : Gain  Gain=Ki
  Gain2 : Gain  Gain=Kp
  Gain3 : Gain  Gain=Ki
  Gain4 : Gain  Gain=Kp
  Mux : Mux  Inputs=2
  Mux2 : Mux  Inputs=3
  Product1 : Product
  Product2 : Product
  Sum : Sum  Inputs=-++
  Sum1 : Sum  Inputs=+++
  Sum2 : Sum  Inputs=|++
  Sum3 : Sum  Inputs=|+-
  Sum4 : Sum  Inputs=|++
  Sum5 : Sum  Inputs=|+-
  Terminator : Terminator
  Terminator1 : Terminator
  Terminator2 : Terminator
  Vdq_err : Scope  NumInputPorts=2
  Zero : Constant  Value=0  OutDataTypeStr=Inherit: Inherit via back propagation
  i_dq0_inductor : Outport
  V_dq_output_err : Outport  Port=2
  wires:
  Gain3/1 -> Discrete-Time Integrator/1
  V_dq0_output_ref/1 -> Demux2/1
  i_dq0_load/1 -> Demux1/1
  Demux2/1 -> Sum3/1
  Discrete-Time Integrator1/1 -> Sum2/2
  Gain4/1 -> Sum4/1
  Product2/1 -> Sum1/1
  Sum5/1 -> Mux/2, Vdq_err/2, Gain4/1, Gain3/1
  Mux2/1 -> i_dq0_inductor/1
  Demux/2 -> Sum5/2, Product1/2
  Demux/1 -> Sum3/2, Product2/2
  Sum3/1 -> Mux/1, Vdq_err/1, Gain2/1, Gain1/1
  Demux2/3 -> Terminator/1
  V_dq0_output/1 -> Demux/1
  Sum/1 -> Mux2/1
  Demux1/1 -> Sum/2
  Discrete-Time Integrator/1 -> Sum4/2
  Product1/1 -> Sum/1
  Gain2/1 -> Sum2/1
  Sum2/1 -> Sum/3
  Gain1/1 -> Discrete-Time Integrator1/1
  Sum1/1 -> Mux2/2
  Zero/1 -> Mux2/3
  Sum4/1 -> Sum1/3
  Demux1/2 -> Sum1/2
  Demux2/2 -> Sum5/1
  Demux1/3 -> Terminator1/1
  Demux/3 -> Terminator2/1
  wC/1 -> Product2/1, Product1/1
  Mux/1 -> V_dq_output_err/1

== system completed_microinverter_setup/Grid Feeding//Forming Inverter 2/Inverter PI Power Controller ==
  note: Load current PI controller
  note: Use a feedforward term since we know that
      | Idq0_inductor = Idq0_load + Idq0_capacitor
      |
      | We let Idq0_capacitor be compensated for by the integrator
  note: Don't integrate error when operating in grid forming mode
  note: P-Q to Idq0_load conversion
  note: P=Vrms * Irms cos(theta)
      | P = 1/2 * VI * cos(theta)
      |
      | Since Id = Icos(theta), when locked onto V (the output/grid voltage)
      | V = Vd (When PLL is locked onto the grid)
      |
      | P = 1/2 * Vd * Id
      |
      | Since we have 3 phases
      | P = 3/2 * Vd * Id
      |
      | Therefore for a reference power, we get
      | Id_ref = P * 2/3 * (1/Vd)
      |
      | Likewise for Q = Vrms * Irms * sin(theta)
      | Iq_ref = Q * 2/3 * (1/Vd)
  P_ref : Inport
  Q_ref : Inport  Port=2
  Vd : Inport  Port=3
  I_dq0_load_in : Inport  Port=4
  Grid Connect Signal : Inport  Port=5
  Constant11 : Constant  Value=0
  Demux1 : Demux  Outputs=2
  Discrete-Time Integrator2 : DiscreteIntegrator  SampleTime=Ts  LimitOutput=on  UpperSaturationLimit=100  LowerSaturationLimit=-100  ICPrevOutput=DiscIntNeverNeededParam  ICPrevScaledInput=DiscIntNeverNeededParam
  Divide : Product  Inputs=*/
  Gain1 : Gain  Gain=2/3
  Gain2 : Gain  Gain=Kp
  Gain4 : Gain  Gain=Ki
  Mux : Mux  Inputs=2
  Mux3 : Mux  Inputs=3
  Scope7 : Scope
  Scope9 : Scope
  Sum : Sum  Inputs=+-|
  Sum1 : Sum  Inputs=|++
  Sum2 : Sum  Inputs=|++
  Switch1 : Switch  Criteria=u2 > Threshold  SaturateOnIntegerOverflow=off  InputSameDT=off
  Zero : Constant  Value=0  OutDataTypeStr=Inherit: Inherit via back propagation
  I_dq0_inductor : Outport
  wires:
  Sum/1 -> Switch1/1  "I_dq0_error"
  Zero/1 -> Switch1/3
  Discrete-Time Integrator2/1 -> Sum1/2
  Sum2/1 -> I_dq0_inductor/1
  Gain4/1 -> Discrete-Time Integrator2/1
  Grid Connect Signal/1 -> Switch1/2
  Gain1/1 -> Divide/1
  Demux1/1 -> Mux3/1  "Id"
  Constant11/1 -> Mux3/3
  Demux1/2 -> Mux3/2  "Iq"
  Divide/1 -> Demux1/1
  Q_ref/1 -> Mux/2
  P_ref/1 -> Mux/1
  Vd/1 -> Divide/2
  Mux/1 -> Gain1/1
  Mux3/1 -> Scope9/1, Sum/1, Sum2/1  "I_dq0_load_ref"
  Switch1/1 -> Scope7/1, Gain4/1, Gain2/1
  Gain2/1 -> Sum1/1
  Sum1/1 -> Sum2/2  "I_dq0_adjust"
  I_dq0_load_in/1 -> Sum/2

== system completed_microinverter_setup/Grid Feeding//Forming Inverter 2/PLL ==
  Vabc : Inport
  Constant1 : Constant  Value=f_center
  Delay : Delay  DelayLength=1  SampleTime=Ts
  Demux : Demux  Outputs=3
  Divide : Product  Inputs=*/
  Gain : Gain  Gain=2*pi
  Gain3 : Gain  Gain=2/3
  PI Controller : Subsystem
  Saturation : Saturate  UpperLimit=2*pi*4.8  LowerLimit=-2*pi*4.8
  Scope{,1..3} (4 alike) : Scope
  Sqrt : Sqrt
  Square : Math  Operator=square
  Sum of Elements : Sum  Inputs=+
  Terminator : Terminator
  Terminator1 : Terminator
  Transform : Subsystem
  Zero-Order Hold : ZeroOrderHold  SampleTime=Ts
  abc to dq0 : spsabctodq0Lib/abc to dq0  Alignment=Aligned with phase A axis
  Amp_est : Outport
  w_est : Outport  Port=2
  wt : Outport  Port=3
  Vdq0 : Outport  Port=4
  wires:
  Square/1 -> Sum of Elements/1
  Sum of Elements/1 -> Gain3/1
  Gain3/1 -> Sqrt/1
  Constant1/1 -> Transform/2(f_center)
  Divide/1 -> Scope1/1, PI Controller/1(Vq)
  PI Controller/1(U) -> Saturation/1
  Sqrt/1 -> Divide/2, Scope/1, Amp_est/1
  Transform/2(f_out) -> Scope2/1, Gain/1
  Transform/1(wt) -> abc to dq0/2, wt/1
  Zero-Order Hold/1 -> abc to dq0/1, Square/1
  Saturation/1 -> Delay/1
  Delay/1 -> Transform/1(U)
  Vabc/1 -> Zero-Order Hold/1
  abc to dq0/1 -> Scope3/1, Vdq0/1, Demux/1
  Demux/2 -> Divide/1
  Gain/1 -> w_est/1
  Demux/3 -> Terminator/1
  Demux/1 -> Terminator1/1
